simulink model "ROPOD_4Wheel_TdistZMPC_cntr"  (R2017b)
settings: Solver=FixedStepAuto  StartTime=0.0  StopTime=Inf  FixedStep=Ts  RelTol=1e-3
PreLoadFcn:
  | cd /home/robocup/RoPod/Force_dist_ZMPC_ROS
  | init_model
InitFcn:
  | cd /home/robocup/RoPod/Force_dist_ZMPC_ROS
  | init_model
values from neighbouring files (symbols this model uses):
  b_cx = 36.5    [RoPod_parameters.mat]
  b_cy = 36.5    [RoPod_parameters.mat]
  Fd_max = 70    [RoPod_parameters.mat]
  Fd_min = 20    [RoPod_parameters.mat]
  FFtheta_intia = 0    [init_model.m]
  FFxy_mass = 80    [init_model.m]
  Fr_max = 100    [RoPod_parameters.mat]
  Fr_min = -100    [RoPod_parameters.mat]
  k_cx = 1713    [RoPod_parameters.mat]
  k_cy = 4489    [RoPod_parameters.mat]
  max_hw_tau = 7.0    (= 7)    [init_model.m]
  Nwheels = 4    [init_model.m]
  pivot_offs_sws = [2.21 1.873 2.001 3.508]    [init_model.m]
  SW_COM1_ENABLE1 = hex2dec('0001')    [init_model.m]
  SW_COM1_ENABLE2 = hex2dec('0002')    [init_model.m]
  SW_COM1_MODE_TORQUE = bitshift(hex2dec('0000'),2)    [init_model.m]
  SW_COM1_MODE_VELOCITY = bitshift(hex2dec('0002'),2)    [init_model.m]
  SW_COM1_USE_TS = hex2dec('8000')    [init_model.m]
  sw_tau_2_curr = 1/motor_physical_parameters.torqueconstant.value    [init_model.m]
  Taucompfactor = 2.0    (= 2)    [init_model.m]
  Tinit = 1*Tslot    [init_model.m]
  Ts = 0.001    [init_model.m]
  Ts_MPC = 0.001    [init_model.m]
  Tsp = 1    [init_model.m]
  xA = [1 -1 0 0 0 0 0.0206696424966 -0.0206696424966 0 0 0.0298227588181 -0.0298227588181 ... (4080 elements, 102x40)]    [ZMPCx_parameters.mat]
  xBd_dis = [1.12932348493e-06 0.000225071897401 0 0]    [ZMPCx_parameters.mat]
  xF = [0 0 0 0 0 0 0 0 0 0 0 0 ... (80 elements, 20x4)]    [ZMPCx_parameters.mat]
  xH = [20 0 0 0 0 0 0 0 0 0 0 0 ... (1600 elements, 40x40)]    [ZMPCx_parameters.mat]
  xPhi = [0.995143909015 -0.967809158823 0 0 0.980727027327 -1.91066813489 0 0 0.957042868744 -2.81984596436 0 0 ... (320 elements, 80x4)]    [ZMPCx_parameters.mat]
  xrho = 144000    [ZMPCx_parameters.mat]
  xW = [0 0 -4300 4300 0 0 -4211.12053726 4211.12053726 0 0 -4082.88267435 4082.88267435 ... (328 elements, 82x4)]    [ZMPCx_parameters.mat]
  yA = [1 -1 0 0 0 0 0.0146537039222 -0.0146537039222 0 0 0.0255124036215 -0.0255124036215 ... (4080 elements, 102x40)]    [ZMPCy_parameters.mat]
  yBd_dis = [1.24492522358e-06 0.000248362591603 0 0]    [ZMPCy_parameters.mat]
  yF = [0.00191047141222 0.00156448969707 0.00119761396088 0.000813779538874 0.00041715000072 1.20724055612e-05 -0.00039696993291 -0.000805406662726 -0.00120863105559 -0.00160205155743 -0.00198114365531 -0.00234150147928 ... (80 elements, 20x4)]    [ZMPCy_parameters.mat]
  yH = [2.00000002801 0 2.31602594113e-08 0 1.80085634996e-08 0 1.26053094289e-08 0 7.00898668547e-09 0 1.2808124932e-09 0 ... (1600 elements, 40x40)]    [ZMPCy_parameters.mat]
  yPhi = [0.994411530671 -1.11489967371 0 0 0.977778317439 -2.20691845877 0 0 0.950389393786 -3.2640842851 0 0 ... (320 elements, 80x4)]    [ZMPCy_parameters.mat]
  yrho = 10000    [ZMPCy_parameters.mat]
  yW = [0 0 -4489 4489 0 0 -4423.21952309 4423.21952309 0 0 -4308.69434324 4308.69434324 ... (328 elements, 82x4)]    [ZMPCy_parameters.mat]
undefined symbols (not defined in the file or in its folder): DiscIntNeverNeededParam, Pose, ropod_kinmodel_param, Twist, Wrench
libraries: cstblocks x85, robotlib x60, simulink x41, SOEM_EtherCAT_Lib x5, robotcorelib x1
(part 1 of 6)
PreSaveFcn:
  | cd /home/robocup/RoPod/Force_dist_ZMPC_ROS
  | init_model
settings Model: Creator=cesar  LastModifiedBy=root
settings OptimizationCC: PassReuseOutputArgsAs=Individual arguments  MaxStackSize=64
settings DebuggingCC: ParameterTunabilityLossMsg=error
settings HardwareCC: ProdBitPerLong=64  ProdHWDeviceType=Intel->x86-64 (Linux 64)  TargetBitPerLong=64  TargetBitPerPointer=64  TargetBitPerSizeT=64  TargetBitPerPtrDiffT=64  TargetLargestAtomicFloat=Float  TargetIntDivRoundTo=Zero  TargetEndianess=LittleEndian  TargetWordSize=64  TargetHWDeviceType=Intel->x86-64 (Linux 64)
settings SFSimCC: MATLABDynamicMemAlloc=off
settings RTWCC: SystemTargetFile=ert.tlc  HardwareBoard=Robot Operating System (ROS)  TemplateMakefile=ert_default_tmf  GenerateReport=on  RTWVerbose=off  CustomInclude=/usr/local/include/soem  CustomLibrary=/usr/local/lib/libsoem.so  Toolchain=Catkin  BuildConfiguration=Faster Runs  IncludeHyperlinkInReport=on  LaunchReport=on  TargetLang=C++  GenerateTraceInfo=on  GenerateTraceReport=on  GenerateTraceReportSl=on  GenerateTraceReportSf=on  GenerateTraceReportEml=on
settings CodeAppCC: ForceParamTrailComments=on  IgnoreCustomStorageClasses=off  OperatorAnnotations=on  SimulinkDataObjDesc=on  SFDataObjDesc=on  InsertBlockDesc=on
settings ERTTargetCC: SupportNonInlinedSFcns=on  SupportVariableSizeSignals=on

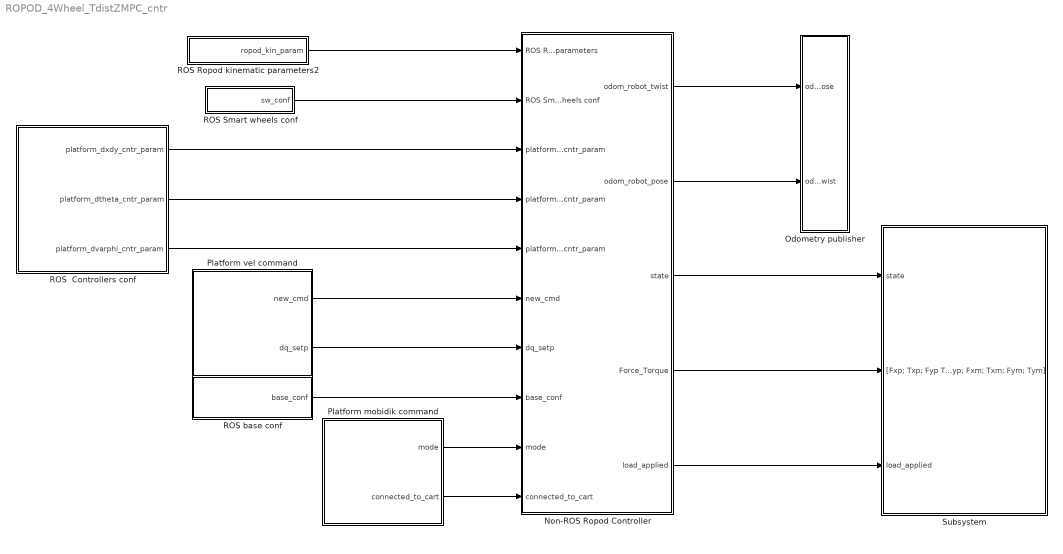
== system ROPOD_4Wheel_TdistZMPC_cntr ==
  Non-ROS Ropod Controller : Subsystem
  Odometry publisher : Subsystem
  Platform mobidik command : Subsystem
  Platform vel command : Subsystem
  ROS  Controllers conf : Subsystem
  ROS Ropod kinematic parameters2 : Subsystem
  ROS Smart wheels conf : Subsystem
  ROS base conf : Subsystem
  Subsystem : Subsystem
  wires:
  ROS Ropod kinematic parameters2/1(ropod_kin_param) -> Non-ROS Ropod Controller/1(ROS Ropod kinematic parameters)
  ROS Smart wheels conf/1(sw_conf) -> Non-ROS Ropod Controller/2(ROS Smart wheels conf)
  ROS  Controllers conf/1(platform_dxdy_cntr_param) -> Non-ROS Ropod Controller/3(platform_dxdy_cntr_param)
  ROS  Controllers conf/2(platform_dtheta_cntr_param) -> Non-ROS Ropod Controller/4(platform_dtheta_cntr_param)
  ROS  Controllers conf/3(platform_dvarphi_cntr_param) -> Non-ROS Ropod Controller/5(platform_dvarphi_cntr_param)
  Platform vel command/1(new_cmd) -> Non-ROS Ropod Controller/6(new_cmd)
  Platform vel command/2(dq_setp) -> Non-ROS Ropod Controller/7(dq_setp)
  ROS base conf/1(base_conf) -> Non-ROS Ropod Controller/8(base_conf)
  Non-ROS Ropod Controller/1(odom_robot_twist) -> Odometry publisher/1(odom_pose)
  Non-ROS Ropod Controller/2(odom_robot_pose) -> Odometry publisher/2(odom_twist)
  Non-ROS Ropod Controller/3(state) -> Subsystem/1(state)
  Non-ROS Ropod Controller/4(Force_Torque) -> Subsystem/2("[Fxp; Txp; Fyp Typ; Fxm; Txm; Fym; Tym] ")
  Platform mobidik command/1(mode) -> Non-ROS Ropod Controller/9(mode)
  Platform mobidik command/2(connected_to_cart) -> Non-ROS Ropod Controller/10(connected_to_cart)
  Non-ROS Ropod Controller/5(load_applied) -> Subsystem/3(load_applied)

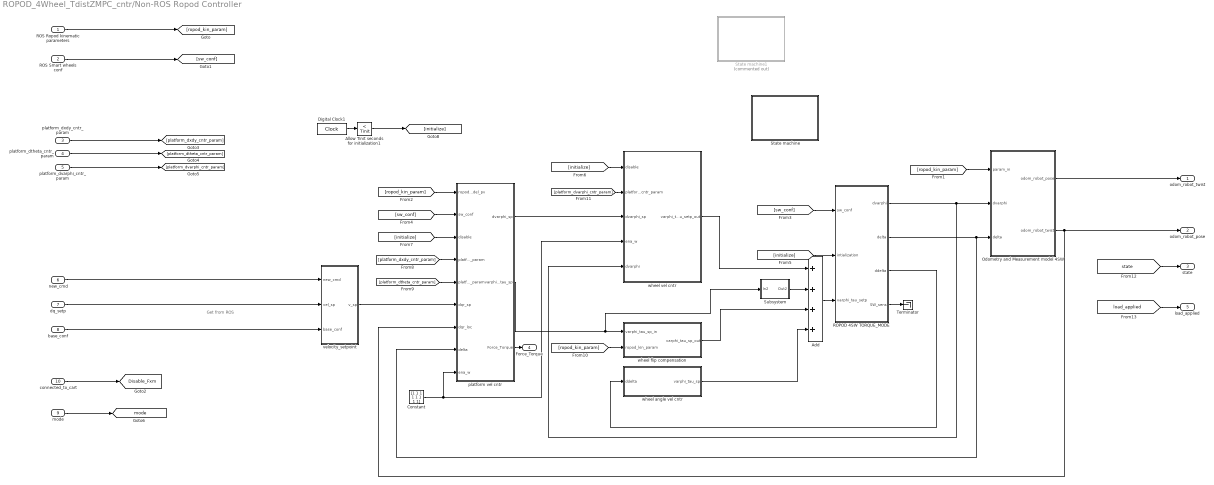
== system ROPOD_4Wheel_TdistZMPC_cntr/Non-ROS Ropod Controller ==
  note: Get from ROS
  ROS Ropod kinematic parameters : Inport
  ROS Smart wheels conf : Inport  Port=2
  platform_dxdy_cntr_param : Inport  Port=3
  platform_dtheta_cntr_param : Inport  Port=4
  platform_dvarphi_cntr_param : Inport  Port=5
  new_cmd : Inport  Port=6
  dq_setp : Inport  Port=7
  base_conf : Inport  Port=8
  mode : Inport  Port=9
  connected_to_cart : Inport  Port=10
  Add : Sum  Inputs=++++
  Allow Tinit seconds for initialization1 : simulink/Logic and Bit Operations/Compare To Constant  relop=<  const=Tinit  OutDataTypeStr=boolean
  Constant : Constant  Value=[1 1 1 1 1 1 1 1]
  Digital Clock1 : DigitalClock  SampleTime=Ts
  Odometry and Measurement model 4SW : Subsystem
  ROPOD 4SW TORQUE_MODE : Subsystem
  State machine : Subsystem
  State machine1 : Subsystem  Commented=on
  Subsystem : Subsystem
  Terminator : Terminator
  platform vel cntr : Subsystem
  velocity_setpoint : Subsystem
  wheel angle vel cntr : Subsystem
  wheel flip compensation : Subsystem
  wheel vel cntr : Subsystem
  odom_robot_twist : Outport
  odom_robot_pose : Outport  Port=2
  state : Outport  Port=3
  Force_Torque : Outport  Port=4
  load_applied : Outport  Port=5
  tag scope: Disable_Fxm=global, mode=global
  wires:
  [sw_conf] -> ROPOD 4SW TORQUE_MODE/1(sw_conf)
  ROPOD 4SW TORQUE_MODE/3(ddelta) -> wheel angle vel cntr/1(ddelta)
  [initialize] -> wheel vel cntr/1(disable)
  base_conf/1 -> velocity_setpoint/3(base_conf)
  Digital Clock1/1 -> Allow Tinit seconds for initialization1/1
  [sw_conf] -> platform vel cntr/2(sw_conf)
  [platform_dvarphi_cntr_param] -> wheel vel cntr/2(platform_dxdy_cntr_param)
  wheel angle vel cntr/1(varphi_tau_sp) -> Add/4
  ROPOD 4SW TORQUE_MODE/2(delta) -> Odometry and Measurement model 4SW/3(delta), platform vel cntr/8(delta)
  [platform_dtheta_cntr_param] -> platform vel cntr/5(platform_dtheta_cntr_param)
  platform vel cntr/2(varphi_tau_sp) -> Subsystem/1(In2), wheel flip compensation/1(varphi_tau_sp_in)
  Add/1 -> ROPOD 4SW TORQUE_MODE/3(varphi_tau_setp)
  [platform_dxdy_cntr_param] -> platform vel cntr/4(platform_dxdy_cntr_param)
  [ropod_kin_param] -> platform vel cntr/1(ropod_kinmodel_pv)
  velocity_setpoint/1(v_sp) -> platform vel cntr/6(dqr_sp)
  wheel flip compensation/1(varphi_tau_sp_out) -> Add/3
  ROS Smart wheels conf/1 -> [sw_conf]
  platform_dvarphi_cntr_param/1 -> [platform_dvarphi_cntr_param]
  Odometry and Measurement model 4SW/1(odom_robot_pose) -> odom_robot_twist/1
  [ropod_kin_param] -> Odometry and Measurement model 4SW/1(param_in)
  [initialize] -> platform vel cntr/3(disable)
  ROPOD 4SW TORQUE_MODE/4(SW_sens) -> Terminator/1
  platform_dxdy_cntr_param/1 -> [platform_dxdy_cntr_param]
  ROS Ropod kinematic parameters/1 -> [ropod_kin_param]
  [initialize] -> ROPOD 4SW TORQUE_MODE/2(intialization)
  [ropod_kin_param] -> wheel flip compensation/2(ropod_kin_param)
  platform vel cntr/1(dvarphi_sp) -> wheel vel cntr/3(dvarphi_sp)
  Odometry and Measurement model 4SW/2(odom_robot_twist) -> odom_robot_pose/1, platform vel cntr/7(dqr_loc)
  ROPOD 4SW TORQUE_MODE/1(dvarphi) -> Odometry and Measurement model 4SW/2(dvarphi), wheel vel cntr/5(dvarphi)
  platform_dtheta_cntr_param/1 -> [platform_dtheta_cntr_param]
  new_cmd/1 -> velocity_setpoint/1(new_cmd)
  dq_setp/1 -> velocity_setpoint/2(vel_sp)
  Constant/1 -> wheel vel cntr/4(ena_w), platform vel cntr/9(ena_w)
  Allow Tinit seconds for initialization1/1 -> [initialize]
  wheel vel cntr/1(varphi_tau_setp_out) -> Add/1
  Subsystem/1(Out2) -> Add/2
  connected_to_cart/1 -> [Disable_Fxm]
  mode/1 -> [mode]
  [state] -> state/1
  platform vel cntr/3(Force_Torque) -> Force_Torque/1
  [load_applied] -> load_applied/1

== system ROPOD_4Wheel_TdistZMPC_cntr/Odometry publisher ==
  odom_pose : Inport
  odom_twist : Inport  Port=2
  Blank Message : robotlib/Blank Message  SourceLibraryInfo=This block requires Robotics System Toolbox  messageType=nav_msgs/Odometry  SampleTime=-1
      settings: SourceProductBaseCode=RO
  Bus Assignment : BusAssignment  AssignedSignals=Pose.Pose.Position.X,Pose.Pose.Position.Y,Pose.Pose.Position.Z,Pose.Pose.Orientation.W,Pose.Pose.Orientation.X,Pose.Pose.Orientation.Y,Pose.Pose.Orientation.Z,Twist.Twist.Linear.X,Twist.Twist.Linear.Y,Twist.Twist.Linear.Z,Twist.Twist.Angular.X,Twist.Twist.Angular.Y,Twist.Twist.Angular.Z
  Constant{,1..5} (6 alike) : Constant  Value=0
  Coordinate Transformation Conversion : robotcorelib/Coordinate Transformation Conversion  InputRepresentation=Euler Angles  InputEulerSequence=XYZ  ShowTrVecInputPort=on  OutputRepresentation=Quaternion  OutputEulerSequence=ZYX  ShowTrVecOutputPort=on  SimulateUsing=Code generation
      settings: SourceProductBaseCode=RO
  Demux : Demux  Outputs=3
  Demux1 : Demux
  Demux2 : Demux  Outputs=3
  Mux : Mux  Inputs=3
  Publish : robotlib/Publish  SourceLibraryInfo=This block requires Robotics System Toolbox  topicSource=Specify your own  topic=/odom_incomplete  messageType=nav_msgs/Odometry  messageQueueLength=1
      settings: SourceProductBaseCode=RO
  Rate Transition : RateTransition  OutPortSampleTime=Ts_rost
  wires:
  Demux2/2 -> Bus Assignment/10
  Bus Assignment/1 -> Rate Transition/1
  Constant2/1 -> Mux/2
  Constant3/1 -> Bus Assignment/11
  Constant/1 -> Bus Assignment/4
  Constant4/1 -> Bus Assignment/12
  Demux2/1 -> Bus Assignment/9
  Coordinate Transformation Conversion/1 -> Demux1/1
  Constant5/1 -> Bus Assignment/13
  Demux/3 -> Mux/3
  Mux/1 -> Coordinate Transformation Conversion/1
  odom_pose/1 -> Demux/1
  Demux/1 -> Bus Assignment/2
  Constant1/1 -> Mux/1
  odom_twist/1 -> Demux2/1
  Demux/2 -> Bus Assignment/3
  Blank Message/1 -> Bus Assignment/1
  Demux2/3 -> Bus Assignment/14
  Rate Transition/1 -> Publish/1
  Demux1/1 -> Bus Assignment/5
  Demux1/2 -> Bus Assignment/6
  Demux1/3 -> Bus Assignment/7
  Demux1/4 -> Bus Assignment/8

== system ROPOD_4Wheel_TdistZMPC_cntr/Platform mobidik command ==
  Bus Selector : BusSelector  OutputSignals=Data
  Bus Selector1 : BusSelector  OutputSignals=Data
  Subscribe1 : robotlib/Subscribe  SourceLibraryInfo=This block requires Robotics System Toolbox  topicSource=Specify your own  topic=/ropod/Set_LLCmode  messageType=std_msgs/UInt16  sampleTime=Ts_rost  messageQueueLength=5
      settings: SourceProductBaseCode=RO
  Subscribe2 : robotlib/Subscribe  SourceLibraryInfo=This block requires Robotics System Toolbox  topicSource=Specify your own  topic=/route_navigation/set_load_attached  messageType=std_msgs/Bool  sampleTime=Ts_rost  messageQueueLength=5
      settings: SourceProductBaseCode=RO
  Terminator : Terminator
  Terminator1 : Terminator
  mode : Outport
  connected_to_cart : Outport  Port=2
  wires:
  Subscribe2/2 -> Bus Selector/1
  Subscribe1/1 -> Terminator/1
  Subscribe2/1 -> Terminator1/1
  Bus Selector/1 -> connected_to_cart/1  "<Data>"
  Subscribe1/2 -> Bus Selector1/1
  Bus Selector1/1 -> mode/1  "<Data>"

== system ROPOD_4Wheel_TdistZMPC_cntr/Platform vel command ==
  Bus Selector : BusSelector  OutputSignals=Linear.X,Linear.Y,Angular.Z
  Mux : Mux  Inputs=3.
  Subscribe1 : robotlib/Subscribe  SourceLibraryInfo=This block requires Robotics System Toolbox  topicSource=Specify your own  topic=/cmd_vel  messageType=geometry_msgs/Twist  sampleTime=Ts_rost  messageQueueLength=5
      settings: SourceProductBaseCode=RO
  new_cmd : Outport
  dq_setp : Outport  Port=2
  wires:
  Subscribe1/1 -> new_cmd/1
  Subscribe1/2 -> Bus Selector/1
  Bus Selector/1 -> Mux/1  "<X>"
  Bus Selector/2 -> Mux/2  "<Y>"
  Bus Selector/3 -> Mux/3  "<Z>"
  Mux/1 -> dq_setp/1

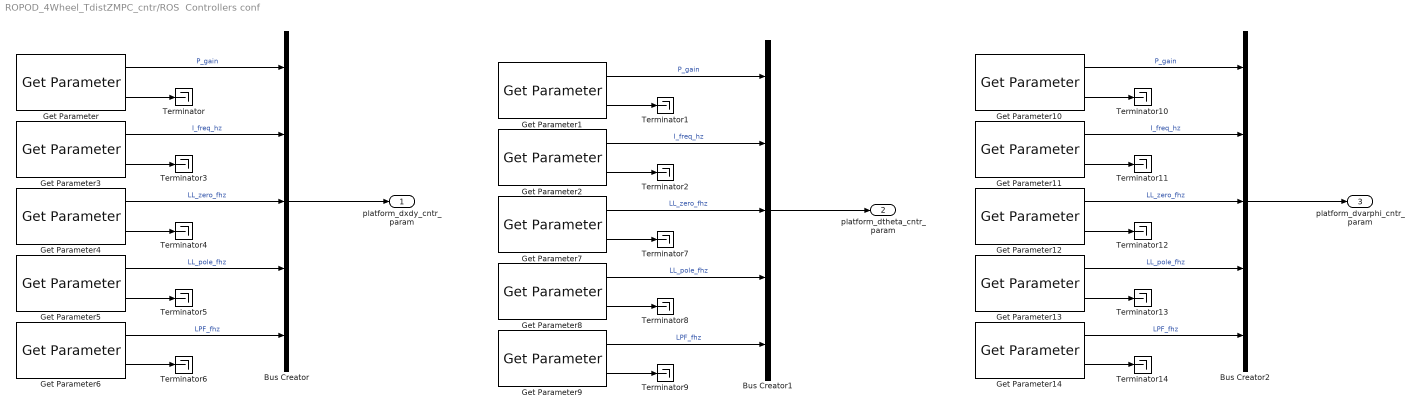
== system ROPOD_4Wheel_TdistZMPC_cntr/ROS  Controllers conf ==
  Bus Creator : BusCreator  Inputs=5
  Bus Creator1 : BusCreator  Inputs=5
  Bus Creator2 : BusCreator  Inputs=5
  Get Parameter : robotlib/Get Parameter  SourceLibraryInfo=This block requires Robotics System Toolbox  ParameterSource=Specify your own  ParameterName=/platform_dxdy_cntr/Kgain  ParameterType=double  ParameterMaxArrayLength=16  ParameterInitialValue=K_gain_dxdy_cntr  SampleTime=Tsp  ShowErrorCodeOutput=on  ModelName=ROPOD_4Wheel_TdistZMPC_cntr  BlockId=ParamGet_ROPOD_4Wheel_TdistZMPC_cntr_2716
      settings: SourceProductName=Robotics System Toolbox  SourceProductBaseCode=RO
  Get Parameter1 : robotlib/Get Parameter  SourceLibraryInfo=This block requires Robotics System Toolbox  ParameterSource=Specify your own  ParameterName=/platform_dtheta_cntr/Kgain  ParameterType=double  ParameterMaxArrayLength=16  ParameterInitialValue=K_gain_dtheta_cntr  SampleTime=Tsp  ShowErrorCodeOutput=on  ModelName=ROPOD_4Wheel_TdistZMPC_cntr  BlockId=ParamGet_ROPOD_4Wheel_TdistZMPC_cntr_2919
      settings: SourceProductName=Robotics System Toolbox  SourceProductBaseCode=RO
  Get Parameter10 : robotlib/Get Parameter  SourceLibraryInfo=This block requires Robotics System Toolbox  ParameterSource=Specify your own  ParameterName=/platform_dvarphi_cntr/Kgain  ParameterType=double  ParameterMaxArrayLength=16  ParameterInitialValue=K_gain_dvarphi_cntr  SampleTime=Tsp  ShowErrorCodeOutput=on  ModelName=ROPOD_4Wheel_TdistZMPC_cntr  BlockId=ParamGet_ROPOD_4Wheel_TdistZMPC_cntr_2931
      settings: SourceProductName=Robotics System Toolbox  SourceProductBaseCode=RO
  Get Parameter11 : robotlib/Get Parameter  SourceLibraryInfo=This block requires Robotics System Toolbox  ParameterSource=Specify your own  ParameterName=/platform_dvarphi_cntr/I_fhz  ParameterType=double  ParameterMaxArrayLength=16  ParameterInitialValue=I_fhz_dvarphi_cntr  SampleTime=Tsp  ShowErrorCodeOutput=on  ModelName=ROPOD_4Wheel_TdistZMPC_cntr  BlockId=ParamGet_ROPOD_4Wheel_TdistZMPC_cntr_2932
      settings: SourceProductName=Robotics System Toolbox  SourceProductBaseCode=RO
  Get Parameter12 : robotlib/Get Parameter  SourceLibraryInfo=This block requires Robotics System Toolbox  ParameterSource=Specify your own  ParameterName=/platform_dvarphi_cntr/LL_wz_fhz  ParameterType=double  ParameterMaxArrayLength=16  ParameterInitialValue=LL_wz_fhz_dvarphi_cntr  SampleTime=Tsp  ShowErrorCodeOutput=on  ModelName=ROPOD_4Wheel_TdistZMPC_cntr  BlockId=ParamGet_ROPOD_4Wheel_TdistZMPC_cntr_2933
      settings: SourceProductName=Robotics System Toolbox  SourceProductBaseCode=RO
  Get Parameter13 : robotlib/Get Parameter  SourceLibraryInfo=This block requires Robotics System Toolbox  ParameterSource=Specify your own  ParameterName=/platform_dvarphi_cntr/LL_wp_fhz  ParameterType=double  ParameterMaxArrayLength=16  ParameterInitialValue=LL_wp_fhz_dvarphi_cntr  SampleTime=Tsp  ShowErrorCodeOutput=on  ModelName=ROPOD_4Wheel_TdistZMPC_cntr  BlockId=ParamGet_ROPOD_4Wheel_TdistZMPC_cntr_2934
      settings: SourceProductName=Robotics System Toolbox  SourceProductBaseCode=RO
  Get Parameter14 : robotlib/Get Parameter  SourceLibraryInfo=This block requires Robotics System Toolbox  ParameterSource=Specify your own  ParameterName=/platform_dvarphi_cntr/LPF_fhz  ParameterType=double  ParameterMaxArrayLength=16  ParameterInitialValue=LPF_fhz_dvarphi_cntr  SampleTime=Tsp  ShowErrorCodeOutput=on  ModelName=ROPOD_4Wheel_TdistZMPC_cntr  BlockId=ParamGet_ROPOD_4Wheel_TdistZMPC_cntr_2935
      settings: SourceProductName=Robotics System Toolbox  SourceProductBaseCode=RO
  Get Parameter2 : robotlib/Get Parameter  SourceLibraryInfo=This block requires Robotics System Toolbox  ParameterSource=Specify your own  ParameterName=/platform_dtheta_cntr/I_fhz  ParameterType=double  ParameterMaxArrayLength=16  ParameterInitialValue=I_fhz_dtheta_cntr  SampleTime=Tsp  ShowErrorCodeOutput=on  ModelName=ROPOD_4Wheel_TdistZMPC_cntr  BlockId=ParamGet_ROPOD_4Wheel_TdistZMPC_cntr_2920
      settings: SourceProductName=Robotics System Toolbox  SourceProductBaseCode=RO
  Get Parameter3 : robotlib/Get Parameter  SourceLibraryInfo=This block requires Robotics System Toolbox  ParameterSource=Specify your own  ParameterName=/platform_dxdy_cntr/I_fhz  ParameterType=double  ParameterMaxArrayLength=16  ParameterInitialValue=I_fhz_dxdy_cntr  SampleTime=Tsp  ShowErrorCodeOutput=on  ModelName=ROPOD_4Wheel_TdistZMPC_cntr  BlockId=ParamGet_ROPOD_4Wheel_TdistZMPC_cntr_2898
      settings: SourceProductName=Robotics System Toolbox  SourceProductBaseCode=RO
  Get Parameter4 : robotlib/Get Parameter  SourceLibraryInfo=This block requires Robotics System Toolbox  ParameterSource=Specify your own  ParameterName=/platform_dxdy_cntr/LL_wz_fhz  ParameterType=double  ParameterMaxArrayLength=16  ParameterInitialValue=LL_wz_fhz_dxdy_cntr  SampleTime=Tsp  ShowErrorCodeOutput=on  ModelName=ROPOD_4Wheel_TdistZMPC_cntr  BlockId=ParamGet_ROPOD_4Wheel_TdistZMPC_cntr_2900
      settings: SourceProductName=Robotics System Toolbox  SourceProductBaseCode=RO
  Get Parameter5 : robotlib/Get Parameter  SourceLibraryInfo=This block requires Robotics System Toolbox  ParameterSource=Specify your own  ParameterName=/platform_dxdy_cntr/LL_wp_fhz  ParameterType=double  ParameterMaxArrayLength=16  ParameterInitialValue=LL_wp_fhz_dxdy_cntr  SampleTime=Tsp  ShowErrorCodeOutput=on  ModelName=ROPOD_4Wheel_TdistZMPC_cntr  BlockId=ParamGet_ROPOD_4Wheel_TdistZMPC_cntr_2902
      settings: SourceProductName=Robotics System Toolbox  SourceProductBaseCode=RO
  Get Parameter6 : robotlib/Get Parameter  SourceLibraryInfo=This block requires Robotics System Toolbox  ParameterSource=Specify your own  ParameterName=/platform_dxdy_cntr/LPF_fhz  ParameterType=double  ParameterMaxArrayLength=16  ParameterInitialValue=LPF_fhz_dxdy_cntr  SampleTime=Tsp  ShowErrorCodeOutput=on  ModelName=ROPOD_4Wheel_TdistZMPC_cntr  BlockId=ParamGet_ROPOD_4Wheel_TdistZMPC_cntr_2903
      settings: SourceProductName=Robotics System Toolbox  SourceProductBaseCode=RO
  Get Parameter7 : robotlib/Get Parameter  SourceLibraryInfo=This block requires Robotics System Toolbox  ParameterSource=Specify your own  ParameterName=/platform_dtheta_cntr/LL_wz_fhz  ParameterType=double  ParameterMaxArrayLength=16  ParameterInitialValue=LL_wz_fhz_dtheta_cntr  SampleTime=Tsp  ShowErrorCodeOutput=on  ModelName=ROPOD_4Wheel_TdistZMPC_cntr  BlockId=ParamGet_ROPOD_4Wheel_TdistZMPC_cntr_2921
      settings: SourceProductName=Robotics System Toolbox  SourceProductBaseCode=RO
  Get Parameter8 : robotlib/Get Parameter  SourceLibraryInfo=This block requires Robotics System Toolbox  ParameterSource=Specify your own  ParameterName=/platform_dtheta_cntr/LL_wp_fhz  ParameterType=double  ParameterMaxArrayLength=16  ParameterInitialValue=LL_wp_fhz_dtheta_cntr  SampleTime=Tsp  ShowErrorCodeOutput=on  ModelName=ROPOD_4Wheel_TdistZMPC_cntr  BlockId=ParamGet_ROPOD_4Wheel_TdistZMPC_cntr_2922
      settings: SourceProductName=Robotics System Toolbox  SourceProductBaseCode=RO
  Get Parameter9 : robotlib/Get Parameter  SourceLibraryInfo=This block requires Robotics System Toolbox  ParameterSource=Specify your own  ParameterName=/platform_dtheta_cntr/LPF_fhz  ParameterType=double  ParameterMaxArrayLength=16  ParameterInitialValue=LPF_fhz_dtheta_cntr  SampleTime=Tsp  ShowErrorCodeOutput=on  ModelName=ROPOD_4Wheel_TdistZMPC_cntr  BlockId=ParamGet_ROPOD_4Wheel_TdistZMPC_cntr_2923
      settings: SourceProductName=Robotics System Toolbox  SourceProductBaseCode=RO
  Terminator{,1..14} (15 alike) : Terminator
  platform_dxdy_cntr_param : Outport
  platform_dtheta_cntr_param : Outport  Port=2
  platform_dvarphi_cntr_param : Outport  Port=3
  wires:
  Get Parameter/2 -> Terminator/1
  Get Parameter5/1 -> Bus Creator/4  "LL_pole_fhz"
  Get Parameter6/1 -> Bus Creator/5  "LPF_fhz"
  Bus Creator/1 -> platform_dxdy_cntr_param/1
  Get Parameter3/1 -> Bus Creator/2  "I_freq_hz"
  Get Parameter4/1 -> Bus Creator/3  "LL_zero_fhz"
  Get Parameter/1 -> Bus Creator/1  "P_gain"
  Get Parameter3/2 -> Terminator3/1
  Get Parameter4/2 -> Terminator4/1
  Get Parameter5/2 -> Terminator5/1
  Get Parameter6/2 -> Terminator6/1
  Get Parameter8/1 -> Bus Creator1/4  "LL_pole_fhz"
  Get Parameter9/2 -> Terminator9/1
  Get Parameter2/1 -> Bus Creator1/2  "I_freq_hz"
  Get Parameter8/2 -> Terminator8/1
  Bus Creator1/1 -> platform_dtheta_cntr_param/1
  Get Parameter2/2 -> Terminator2/1
  Get Parameter7/1 -> Bus Creator1/3  "LL_zero_fhz"
  Get Parameter7/2 -> Terminator7/1
  Get Parameter1/1 -> Bus Creator1/1  "P_gain"
  Get Parameter1/2 -> Terminator1/1
  Get Parameter9/1 -> Bus Creator1/5  "LPF_fhz"
  Get Parameter10/2 -> Terminator10/1
  Get Parameter13/2 -> Terminator13/1
  Get Parameter14/2 -> Terminator14/1
  Get Parameter11/1 -> Bus Creator2/2  "I_freq_hz"
  Get Parameter10/1 -> Bus Creator2/1  "P_gain"
  Get Parameter11/2 -> Terminator11/1
  Get Parameter13/1 -> Bus Creator2/4  "LL_pole_fhz"
  Bus Creator2/1 -> platform_dvarphi_cntr_param/1
  Get Parameter12/2 -> Terminator12/1
  Get Parameter12/1 -> Bus Creator2/3  "LL_zero_fhz"
  Get Parameter14/1 -> Bus Creator2/5  "LPF_fhz"

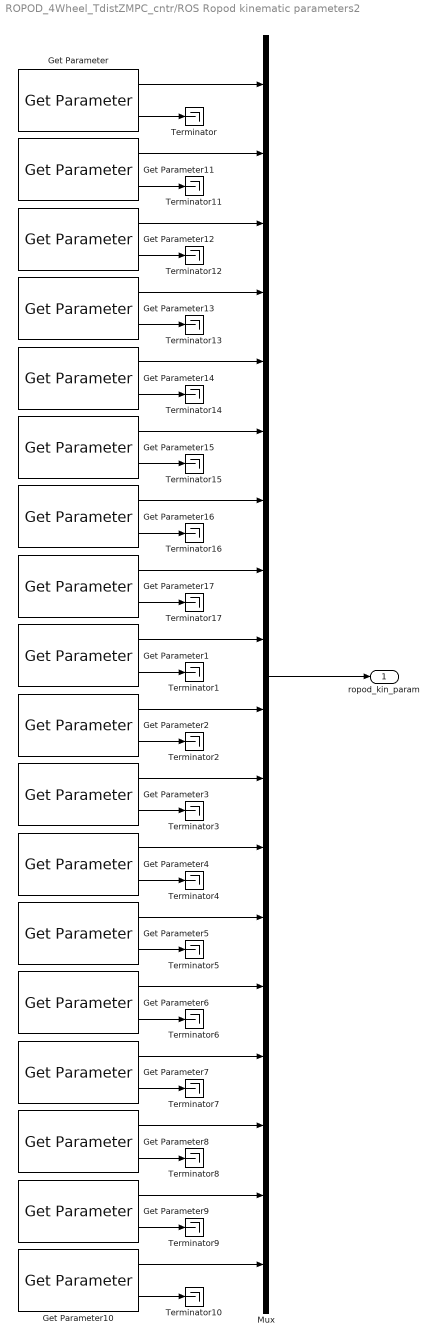
== system ROPOD_4Wheel_TdistZMPC_cntr/ROS Ropod kinematic parameters2 ==
  Get Parameter : robotlib/Get Parameter  SourceLibraryInfo=This block requires Robotics System Toolbox  ParameterSource=Specify your own  ParameterName=/base_kin_model/r_wL_SW1  ParameterType=double  ParameterMaxArrayLength=16  ParameterInitialValue=ropod_kinmodel_param.r_w(1)  SampleTime=Tsp  ShowErrorCodeOutput=on  ModelName=ROPOD_4Wheel_TdistZMPC_cntr  BlockId=ParamGet_ROPOD_4Wheel_TdistZMPC_cntr_2173
      settings: SourceProductName=Robotics System Toolbox  SourceProductBaseCode=RO
  Get Parameter1 : robotlib/Get Parameter  SourceLibraryInfo=This block requires Robotics System Toolbox  ParameterSource=Specify your own  ParameterName=/base_kin_model/s_w  ParameterType=double  ParameterMaxArrayLength=16  ParameterInitialValue=ropod_kinmodel_param.s_w  SampleTime=Tsp  ShowErrorCodeOutput=on  ModelName=ROPOD_4Wheel_TdistZMPC_cntr  BlockId=ParamGet_ROPOD_4Wheel_TdistZMPC_cntr_2174
      settings: SourceProductName=Robotics System Toolbox  SourceProductBaseCode=RO
  Get Parameter10 : robotlib/Get Parameter  SourceLibraryInfo=This block requires Robotics System Toolbox  ParameterSource=Specify your own  ParameterName=/base_kin_model/ypos_SW4  ParameterType=double  ParameterMaxArrayLength=16  ParameterInitialValue=ropod_kinmodel_param.C_SW(8)  SampleTime=Tsp  ShowErrorCodeOutput=on  ModelName=ROPOD_4Wheel_TdistZMPC_cntr  BlockId=ParamGet_ROPOD_4Wheel_TdistZMPC_cntr_2175
      settings: SourceProductName=Robotics System Toolbox  SourceProductBaseCode=RO
  Get Parameter11 : robotlib/Get Parameter  SourceLibraryInfo=This block requires Robotics System Toolbox  ParameterSource=Specify your own  ParameterName=/base_kin_model/r_wR_SW1  ParameterType=double  ParameterMaxArrayLength=16  ParameterInitialValue=ropod_kinmodel_param.r_w(2)  SampleTime=Tsp  ShowErrorCodeOutput=on  ModelName=ROPOD_4Wheel_TdistZMPC_cntr  BlockId=ParamGet_ROPOD_4Wheel_TdistZMPC_cntr_2176
      settings: SourceProductName=Robotics System Toolbox  SourceProductBaseCode=RO
  Get Parameter12 : robotlib/Get Parameter  SourceLibraryInfo=This block requires Robotics System Toolbox  ParameterSource=Specify your own  ParameterName=/base_kin_model/r_wL_SW2  ParameterType=double  ParameterMaxArrayLength=16  ParameterInitialValue=ropod_kinmodel_param.r_w(3)  SampleTime=Tsp  ShowErrorCodeOutput=on  ModelName=ROPOD_4Wheel_TdistZMPC_cntr  BlockId=ParamGet_ROPOD_4Wheel_TdistZMPC_cntr_2177
      settings: SourceProductName=Robotics System Toolbox  SourceProductBaseCode=RO
  Get Parameter13 : robotlib/Get Parameter  SourceLibraryInfo=This block requires Robotics System Toolbox  ParameterSource=Specify your own  ParameterName=/base_kin_model/r_wR_SW2  ParameterType=double  ParameterMaxArrayLength=16  ParameterInitialValue=ropod_kinmodel_param.r_w(4)  SampleTime=Tsp  ShowErrorCodeOutput=on  ModelName=ROPOD_4Wheel_TdistZMPC_cntr  BlockId=ParamGet_ROPOD_4Wheel_TdistZMPC_cntr_2178
      settings: SourceProductName=Robotics System Toolbox  SourceProductBaseCode=RO
  Get Parameter14 : robotlib/Get Parameter  SourceLibraryInfo=This block requires Robotics System Toolbox  ParameterSource=Specify your own  ParameterName=/base_kin_model/r_wL_SW3  ParameterType=double  ParameterMaxArrayLength=16  ParameterInitialValue=ropod_kinmodel_param.r_w(5)  SampleTime=Tsp  ShowErrorCodeOutput=on  ModelName=ROPOD_4Wheel_TdistZMPC_cntr  BlockId=ParamGet_ROPOD_4Wheel_TdistZMPC_cntr_2179
      settings: SourceProductName=Robotics System Toolbox  SourceProductBaseCode=RO
  Get Parameter15 : robotlib/Get Parameter  SourceLibraryInfo=This block requires Robotics System Toolbox  ParameterSource=Specify your own  ParameterName=/base_kin_model/r_wR_SW3  ParameterType=double  ParameterMaxArrayLength=16  ParameterInitialValue=ropod_kinmodel_param.r_w(6)  SampleTime=Tsp  ShowErrorCodeOutput=on  ModelName=ROPOD_4Wheel_TdistZMPC_cntr  BlockId=ParamGet_ROPOD_4Wheel_TdistZMPC_cntr_2180
      settings: SourceProductName=Robotics System Toolbox  SourceProductBaseCode=RO
  Get Parameter16 : robotlib/Get Parameter  SourceLibraryInfo=This block requires Robotics System Toolbox  ParameterSource=Specify your own  ParameterName=/base_kin_model/r_wL_SW4  ParameterType=double  ParameterMaxArrayLength=16  ParameterInitialValue=ropod_kinmodel_param.r_w(7)  SampleTime=Tsp  ShowErrorCodeOutput=on  ModelName=ROPOD_4Wheel_TdistZMPC_cntr  BlockId=ParamGet_ROPOD_4Wheel_TdistZMPC_cntr_2181
      settings: SourceProductName=Robotics System Toolbox  SourceProductBaseCode=RO
  Get Parameter17 : robotlib/Get Parameter  SourceLibraryInfo=This block requires Robotics System Toolbox  ParameterSource=Specify your own  ParameterName=/base_kin_model/r_wR_SW4  ParameterType=double  ParameterMaxArrayLength=16  ParameterInitialValue=ropod_kinmodel_param.r_w(8)  SampleTime=Tsp  ShowErrorCodeOutput=on  ModelName=ROPOD_4Wheel_TdistZMPC_cntr  BlockId=ParamGet_ROPOD_4Wheel_TdistZMPC_cntr_2182
      settings: SourceProductName=Robotics System Toolbox  SourceProductBaseCode=RO
  Get Parameter2 : robotlib/Get Parameter  SourceLibraryInfo=This block requires Robotics System Toolbox  ParameterSource=Specify your own  ParameterName=/base_kin_model/d_w  ParameterType=double  ParameterMaxArrayLength=16  ParameterInitialValue=ropod_kinmodel_param.d_w  SampleTime=Tsp  ShowErrorCodeOutput=on  ModelName=ROPOD_4Wheel_TdistZMPC_cntr  BlockId=ParamGet_ROPOD_4Wheel_TdistZMPC_cntr_2183
      settings: SourceProductName=Robotics System Toolbox  SourceProductBaseCode=RO
  Get Parameter3 : robotlib/Get Parameter  SourceLibraryInfo=This block requires Robotics System Toolbox  ParameterSource=Specify your own  ParameterName=/base_kin_model/xpos_SW1  ParameterType=double  ParameterMaxArrayLength=16  ParameterInitialValue=ropod_kinmodel_param.C_SW(1)  SampleTime=Tsp  ShowErrorCodeOutput=on  ModelName=ROPOD_4Wheel_TdistZMPC_cntr  BlockId=ParamGet_ROPOD_4Wheel_TdistZMPC_cntr_2184
      settings: SourceProductName=Robotics System Toolbox  SourceProductBaseCode=RO
  Get Parameter4 : robotlib/Get Parameter  SourceLibraryInfo=This block requires Robotics System Toolbox  ParameterSource=Specify your own  ParameterName=/base_kin_model/ypos_SW1  ParameterType=double  ParameterMaxArrayLength=16  ParameterInitialValue=ropod_kinmodel_param.C_SW(2)  SampleTime=Tsp  ShowErrorCodeOutput=on  ModelName=ROPOD_4Wheel_TdistZMPC_cntr  BlockId=ParamGet_ROPOD_4Wheel_TdistZMPC_cntr_2185
      settings: SourceProductName=Robotics System Toolbox  SourceProductBaseCode=RO
  Get Parameter5 : robotlib/Get Parameter  SourceLibraryInfo=This block requires Robotics System Toolbox  ParameterSource=Specify your own  ParameterName=/base_kin_model/xpos_SW2  ParameterType=double  ParameterMaxArrayLength=16  ParameterInitialValue=ropod_kinmodel_param.C_SW(3)  SampleTime=Tsp  ShowErrorCodeOutput=on  ModelName=ROPOD_4Wheel_TdistZMPC_cntr  BlockId=ParamGet_ROPOD_4Wheel_TdistZMPC_cntr_2186
      settings: SourceProductName=Robotics System Toolbox  SourceProductBaseCode=RO
  Get Parameter6 : robotlib/Get Parameter  SourceLibraryInfo=This block requires Robotics System Toolbox  ParameterSource=Specify your own  ParameterName=/base_kin_model/ypos_SW2  ParameterType=double  ParameterMaxArrayLength=16  ParameterInitialValue=ropod_kinmodel_param.C_SW(4)  SampleTime=Tsp  ShowErrorCodeOutput=on  ModelName=ROPOD_4Wheel_TdistZMPC_cntr  BlockId=ParamGet_ROPOD_4Wheel_TdistZMPC_cntr_2187
      settings: SourceProductName=Robotics System Toolbox  SourceProductBaseCode=RO
  Get Parameter7 : robotlib/Get Parameter  SourceLibraryInfo=This block requires Robotics System Toolbox  ParameterSource=Specify your own  ParameterName=/base_kin_model/xpos_SW3  ParameterType=double  ParameterMaxArrayLength=16  ParameterInitialValue=ropod_kinmodel_param.C_SW(5)  SampleTime=Tsp  ShowErrorCodeOutput=on  ModelName=ROPOD_4Wheel_TdistZMPC_cntr  BlockId=ParamGet_ROPOD_4Wheel_TdistZMPC_cntr_2188
      settings: SourceProductName=Robotics System Toolbox  SourceProductBaseCode=RO
  Get Parameter8 : robotlib/Get Parameter  SourceLibraryInfo=This block requires Robotics System Toolbox  ParameterSource=Specify your own  ParameterName=/base_kin_model/ypos_SW3  ParameterType=double  ParameterMaxArrayLength=16  ParameterInitialValue=ropod_kinmodel_param.C_SW(6)  SampleTime=Tsp  ShowErrorCodeOutput=on  ModelName=ROPOD_4Wheel_TdistZMPC_cntr  BlockId=ParamGet_ROPOD_4Wheel_TdistZMPC_cntr_2189
      settings: SourceProductName=Robotics System Toolbox  SourceProductBaseCode=RO
  Get Parameter9 : robotlib/Get Parameter  SourceLibraryInfo=This block requires Robotics System Toolbox  ParameterSource=Specify your own  ParameterName=/base_kin_model/xpos_SW4  ParameterType=double  ParameterMaxArrayLength=16  ParameterInitialValue=ropod_kinmodel_param.C_SW(7)  SampleTime=Tsp  ShowErrorCodeOutput=on  ModelName=ROPOD_4Wheel_TdistZMPC_cntr  BlockId=ParamGet_ROPOD_4Wheel_TdistZMPC_cntr_2190
      settings: SourceProductName=Robotics System Toolbox  SourceProductBaseCode=RO
  Mux : Mux  Inputs=18
  Terminator{,1..17} (18 alike) : Terminator
  ropod_kin_param : Outport
  wires:
  Mux/1 -> ropod_kin_param/1
  Get Parameter/2 -> Terminator/1
  Get Parameter13/1 -> Mux/4
  Get Parameter15/2 -> Terminator15/1
  Get Parameter14/2 -> Terminator14/1
  Get Parameter16/1 -> Mux/7
  Get Parameter15/1 -> Mux/6
  Get Parameter11/1 -> Mux/2
  Get Parameter11/2 -> Terminator11/1
  Get Parameter16/2 -> Terminator16/1
  Get Parameter12/2 -> Terminator12/1
  Get Parameter12/1 -> Mux/3
  Get Parameter/1 -> Mux/1
  Get Parameter17/2 -> Terminator17/1
  Get Parameter13/2 -> Terminator13/1
  Get Parameter17/1 -> Mux/8
  Get Parameter14/1 -> Mux/5
  Get Parameter2/2 -> Terminator2/1
  Get Parameter2/1 -> Mux/10
  Get Parameter1/1 -> Mux/9
  Get Parameter1/2 -> Terminator1/1
  Get Parameter6/2 -> Terminator6/1
  Get Parameter6/1 -> Mux/14
  Get Parameter3/1 -> Mux/11
  Get Parameter5/2 -> Terminator5/1
  Get Parameter5/1 -> Mux/13
  Get Parameter4/1 -> Mux/12
  Get Parameter3/2 -> Terminator3/1
  Get Parameter4/2 -> Terminator4/1
  Get Parameter10/1 -> Mux/18
  Get Parameter10/2 -> Terminator10/1
  Get Parameter8/2 -> Terminator8/1
  Get Parameter7/2 -> Terminator7/1
  Get Parameter9/2 -> Terminator9/1
  Get Parameter7/1 -> Mux/15
  Get Parameter8/1 -> Mux/16
  Get Parameter9/1 -> Mux/17

== system ROPOD_4Wheel_TdistZMPC_cntr/ROS Smart wheels conf ==
  Bus Creator : BusCreator  Inputs=6
  Get Parameter : robotlib/Get Parameter  SourceLibraryInfo=This block requires Robotics System Toolbox  ParameterSource=Specify your own  ParameterName=/smart_wheels/enable  ParameterType=double  ParameterMaxArrayLength=16  ParameterInitialValue=sw_ini_enable  SampleTime=Tsp  ShowErrorCodeOutput=on  ModelName=ROPOD_4Wheel_TdistZMPC_cntr  BlockId=ParamGet_ROPOD_4Wheel_TdistZMPC_cntr_2213
      settings: SourceProductName=Robotics System Toolbox  SourceProductBaseCode=RO
  Get Parameter1 : robotlib/Get Parameter  SourceLibraryInfo=This block requires Robotics System Toolbox  ParameterSource=Specify your own  ParameterName=/smart_wheels/pivot_offs_sw1  ParameterType=double  ParameterMaxArrayLength=16  ParameterInitialValue=pivot_offs_sws(1)  SampleTime=Tsp  ShowErrorCodeOutput=on  ModelName=ROPOD_4Wheel_TdistZMPC_cntr  BlockId=ParamGet_ROPOD_4Wheel_TdistZMPC_cntr_2214
      settings: SourceProductName=Robotics System Toolbox  SourceProductBaseCode=RO
  Get Parameter2 : robotlib/Get Parameter  SourceLibraryInfo=This block requires Robotics System Toolbox  ParameterSource=Specify your own  ParameterName=/smart_wheels/max_current  ParameterType=double  ParameterMaxArrayLength=16  ParameterInitialValue=max_sw_current  SampleTime=Tsp  ShowErrorCodeOutput=on  ModelName=ROPOD_4Wheel_TdistZMPC_cntr  BlockId=ParamGet_ROPOD_4Wheel_TdistZMPC_cntr_2215
      settings: SourceProductName=Robotics System Toolbox  SourceProductBaseCode=RO
  Get Parameter3 : robotlib/Get Parameter  SourceLibraryInfo=This block requires Robotics System Toolbox  ParameterSource=Specify your own  ParameterName=/smart_wheels/pivot_offs_sw2  ParameterType=double  ParameterMaxArrayLength=16  ParameterInitialValue=pivot_offs_sws(2)  SampleTime=Tsp  ShowErrorCodeOutput=on  ModelName=ROPOD_4Wheel_TdistZMPC_cntr  BlockId=ParamGet_ROPOD_4Wheel_TdistZMPC_cntr_2216
      settings: SourceProductName=Robotics System Toolbox  SourceProductBaseCode=RO
  Get Parameter4 : robotlib/Get Parameter  SourceLibraryInfo=This block requires Robotics System Toolbox  ParameterSource=Specify your own  ParameterName=/smart_wheels/pivot_offs_sw3  ParameterType=double  ParameterMaxArrayLength=16  ParameterInitialValue=pivot_offs_sws(3)  SampleTime=Tsp  ShowErrorCodeOutput=on  ModelName=ROPOD_4Wheel_TdistZMPC_cntr  BlockId=ParamGet_ROPOD_4Wheel_TdistZMPC_cntr_2217
      settings: SourceProductName=Robotics System Toolbox  SourceProductBaseCode=RO
  Get Parameter5 : robotlib/Get Parameter  SourceLibraryInfo=This block requires Robotics System Toolbox  ParameterSource=Specify your own  ParameterName=/smart_wheels/pivot_offs_sw4  ParameterType=double  ParameterMaxArrayLength=16  ParameterInitialValue=pivot_offs_sws(4)  SampleTime=Tsp  ShowErrorCodeOutput=on  ModelName=ROPOD_4Wheel_TdistZMPC_cntr  BlockId=ParamGet_ROPOD_4Wheel_TdistZMPC_cntr_2218
      settings: SourceProductName=Robotics System Toolbox  SourceProductBaseCode=RO
  Terminator{,1..5} (6 alike) : Terminator
  sw_conf : Outport
  wires:
  Get Parameter/2 -> Terminator/1
  Get Parameter/1 -> Bus Creator/1  "enable"
  Bus Creator/1 -> sw_conf/1
  Get Parameter2/2 -> Terminator2/1
  Get Parameter2/1 -> Bus Creator/2  "max_current"
  Get Parameter1/1 -> Bus Creator/3  "pivot_offs_sw1"
  Get Parameter1/2 -> Terminator1/1
  Get Parameter3/2 -> Terminator3/1
  Get Parameter3/1 -> Bus Creator/4  "pivot_offs_sw2"
  Get Parameter4/2 -> Terminator4/1
  Get Parameter4/1 -> Bus Creator/5  "pivot_offs_sw3"
  Get Parameter5/2 -> Terminator5/1
  Get Parameter5/1 -> Bus Creator/6  "pivot_offs_sw4"

== system ROPOD_4Wheel_TdistZMPC_cntr/ROS base conf ==
  Bus Creator : BusCreator  Inputs=4
  Get Parameter : robotlib/Get Parameter  SourceLibraryInfo=This block requires Robotics System Toolbox  ParameterSource=Specify your own  ParameterName=/base_conf/max_acc_xy  ParameterType=double  ParameterMaxArrayLength=16  ParameterInitialValue=max_ropod_acc_xy  SampleTime=Tsp  ShowErrorCodeOutput=on  ModelName=ROPOD_4Wheel_TdistZMPC_cntr  BlockId=ParamGet_ROPOD_4Wheel_TdistZMPC_cntr_2237
      settings: SourceProductName=Robotics System Toolbox  SourceProductBaseCode=RO
  Get Parameter1 : robotlib/Get Parameter  SourceLibraryInfo=This block requires Robotics System Toolbox  ParameterSource=Specify your own  ParameterName=/base_conf/max_vel_xy  ParameterType=double  ParameterMaxArrayLength=16  ParameterInitialValue=max_ropod_vel_xy  SampleTime=Tsp  ShowErrorCodeOutput=on  ModelName=ROPOD_4Wheel_TdistZMPC_cntr  BlockId=ParamGet_ROPOD_4Wheel_TdistZMPC_cntr_2238
      settings: SourceProductName=Robotics System Toolbox  SourceProductBaseCode=RO
  Get Parameter2 : robotlib/Get Parameter  SourceLibraryInfo=This block requires Robotics System Toolbox  ParameterSource=Specify your own  ParameterName=/base_conf/max_acc_theta  ParameterType=double  ParameterMaxArrayLength=16  ParameterInitialValue=max_ropod_acc_theta  SampleTime=Tsp  ShowErrorCodeOutput=on  ModelName=ROPOD_4Wheel_TdistZMPC_cntr  BlockId=ParamGet_ROPOD_4Wheel_TdistZMPC_cntr_2239
      settings: SourceProductName=Robotics System Toolbox  SourceProductBaseCode=RO
  Get Parameter3 : robotlib/Get Parameter  SourceLibraryInfo=This block requires Robotics System Toolbox  ParameterSource=Specify your own  ParameterName=/base_conf/max_vel_theta  ParameterType=double  ParameterMaxArrayLength=16  ParameterInitialValue=max_ropod_vel_theta  SampleTime=Tsp  ShowErrorCodeOutput=on  ModelName=ROPOD_4Wheel_TdistZMPC_cntr  BlockId=ParamGet_ROPOD_4Wheel_TdistZMPC_cntr_2240
      settings: SourceProductName=Robotics System Toolbox  SourceProductBaseCode=RO
  Terminator{,1..3} (4 alike) : Terminator
  base_conf : Outport
  wires:
  Get Parameter/2 -> Terminator/1
  Get Parameter1/2 -> Terminator1/1
  Get Parameter/1 -> Bus Creator/2  "max_acc_xy"
  Get Parameter1/1 -> Bus Creator/1  "max_vel_xy"
  Bus Creator/1 -> base_conf/1
  Get Parameter2/2 -> Terminator2/1
  Get Parameter2/1 -> Bus Creator/4  "max_acc_theta"
  Get Parameter3/1 -> Bus Creator/3  "max_vel_theta"
  Get Parameter3/2 -> Terminator3/1

== system ROPOD_4Wheel_TdistZMPC_cntr/Subsystem ==
  state : Inport
  "[Fxp; Txp; Fyp Typ; Fxm; Txm; Fym; Tym] " : Inport  Port=2
  load_applied : Inport  Port=3
  Demux : Demux  Outputs=8
  Publish : robotlib/Publish  SourceLibraryInfo=This block requires Robotics System Toolbox  topicSource=Specify your own  topic=/ropod/wrench_left  messageType=geometry_msgs/WrenchStamped  messageQueueLength=1
      settings: SourceProductBaseCode=RO
  Publish1 : robotlib/Publish  SourceLibraryInfo=This block requires Robotics System Toolbox  topicSource=Specify your own  topic=/ropod/wrench_front  messageType=geometry_msgs/WrenchStamped  messageQueueLength=1
      settings: SourceProductBaseCode=RO
  Publish2 : robotlib/Publish  SourceLibraryInfo=This block requires Robotics System Toolbox  topicSource=Specify your own  topic=/ropod/wrench_back  messageType=geometry_msgs/WrenchStamped  messageQueueLength=1
      settings: SourceProductBaseCode=RO
  Publish3 : robotlib/Publish  SourceLibraryInfo=This block requires Robotics System Toolbox  topicSource=Specify your own  topic=/ropod/wrench_right  messageType=geometry_msgs/WrenchStamped  messageQueueLength=1
      settings: SourceProductBaseCode=RO
  Publish4 : robotlib/Publish  SourceLibraryInfo=This block requires Robotics System Toolbox  topicSource=Specify your own  topic=/ropod/LLCmode_Applied  messageType=std_msgs/UInt16  messageQueueLength=1
      settings: SourceProductBaseCode=RO
  Publish5 : robotlib/Publish  SourceLibraryInfo=This block requires Robotics System Toolbox  topicSource=Specify your own  topic=/ropod/load_attached_Applied  messageType=std_msgs/Bool  messageQueueLength=1
      settings: SourceProductBaseCode=RO
  Subsystem : Subsystem
  Subsystem1 : Subsystem
  Subsystem2 : Subsystem
  Subsystem3 : Subsystem
  Subsystem4 : Subsystem
  Subsystem5 : Subsystem
  wires:
  "[Fxp; Txp; Fyp Typ; Fxm; Txm; Fym; Tym] "/1 -> Demux/1
  Demux/1 -> Subsystem/1(In1)
  Demux/2 -> Subsystem/2(In2)
  Subsystem/1(Out1) -> Publish1/1
  Demux/3 -> Subsystem1/1(In1)
  Demux/4 -> Subsystem1/2(In2)
  Demux/5 -> Subsystem2/1(In1)
  Demux/6 -> Subsystem2/2(In2)
  Demux/7 -> Subsystem3/1(In1)
  Demux/8 -> Subsystem3/2(In2)
  Subsystem1/1(Out1) -> Publish/1
  Subsystem2/1(Out1) -> Publish2/1
  Subsystem3/1(Out1) -> Publish3/1
  state/1 -> Subsystem4/1(In1)
  Subsystem4/1(Out1) -> Publish4/1
  load_applied/1 -> Subsystem5/1(In1)
  Subsystem5/1(Out1) -> Publish5/1

== system ROPOD_4Wheel_TdistZMPC_cntr/Non-ROS Ropod Controller/Odometry and Measurement model 4SW ==
  note: This output is only useful when using ros
      | This data is fed to /odom/pose
  note: This part is in global coordinates
  note: This part is in local coordinates
  param_in : Inport
  dvarphi : Inport  Port=2
  delta : Inport  Port=3
  Discrete-Time Integrator : DiscreteIntegrator  InitialConditionSetting=State (most efficient)  SampleTime=Ts  ICPrevOutput=DiscIntNeverNeededParam  ICPrevScaledInput=DiscIntNeverNeededParam
  Jqwl_matrix : MATLAB Function  TreatAsAtomicUnit=on
  Product3 : Product  Multiplication=Matrix(*)
  Selector3 : Selector  InputPortWidth=3  IndexOptions=Index vector (dialog)  Indices=3  OutputSizes=1
  Signal Specification : SignalSpecification  Dimensions=[3 1]
  pos_rot_matrix : MATLAB Function  TreatAsAtomicUnit=on
  odom_robot_pose : Outport
  odom_robot_twist : Outport  Port=2
  wires:
  Product3/1 -> Signal Specification/1
  param_in/1 -> Jqwl_matrix/1(ropod_kinmodel_param_vec)
  delta/1 -> Jqwl_matrix/2(delta)
  Jqwl_matrix/1(Jqwl) -> Product3/1
  dvarphi/1 -> Product3/2
  Signal Specification/1 -> pos_rot_matrix/1(dqr_loc), odom_robot_twist/1
  Selector3/1 -> pos_rot_matrix/2(theta_odom)
  pos_rot_matrix/1(dqr_glb) -> Discrete-Time Integrator/1
  Discrete-Time Integrator/1 -> odom_robot_pose/1, Selector3/1

== system ROPOD_4Wheel_TdistZMPC_cntr/Non-ROS Ropod Controller/ROPOD 4SW TORQUE_MODE ==
  sw_conf : Inport
  intialization : Inport  Port=2
  varphi_tau_setp : Inport  Port=3
  Bus Creator : BusCreator  Inputs=4
  Display1 : Display
  ECAT_Interface : SOEM_EtherCAT_Lib/ECAT_Interface  Priority=0  IFINTERFACE=eth0  TS=Ts
      settings: SourceProductName=SOEM_EtherCAT_Lib
  Gain1 : Gain  OutDataTypeStr=double
  Initialization switch : Subsystem
  ROPOD_4Wheel_sens : Subsystem
  ROPOD_4Wheel_torque_cmd : Subsystem
  Smart_Wheel_1 : Subsystem
  Smart_Wheel_2 : Subsystem
  Smart_Wheel_3 : Subsystem
  Smart_Wheel_4 : Subsystem
  Subsystem : Subsystem
  empywheel : Subsystem  Commented=on
  dvarphi : Outport
  delta : Outport  Port=2
  ddelta : Outport  Port=3
  SW_sens : Outport  Port=4
  wires:
  ROPOD_4Wheel_sens/2(delta) -> delta/1
  ROPOD_4Wheel_sens/1(dvarphi) -> dvarphi/1
  ECAT_Interface/1 -> Gain1/1
  Gain1/1 -> Display1/1
  ROPOD_4Wheel_sens/3(ddelta) -> ddelta/1
  ROPOD_4Wheel_torque_cmd/4(SW4_cmd) -> Smart_Wheel_4/1(SW4_cmd)
  ROPOD_4Wheel_torque_cmd/1(SW1_cmd) -> Smart_Wheel_1/1(SW1_cmd)
  ROPOD_4Wheel_torque_cmd/3(SW3_cmd) -> Smart_Wheel_3/1(SW3_cmd)
  sw_conf/1 -> ROPOD_4Wheel_torque_cmd/1(sw_conf), ROPOD_4Wheel_sens/2(sw_conf)
  ROPOD_4Wheel_torque_cmd/2(SW2_cmd) -> Smart_Wheel_2/1(SW2_cmd)
  Smart_Wheel_1/1(SW1_sens) -> Bus Creator/1, ROPOD_4Wheel_sens/3(SW1_sens)  "SW1_sens"
  Smart_Wheel_4/1(SW4_sens) -> ROPOD_4Wheel_sens/6(SW4_sens), Bus Creator/4  "SW4_sens"
  Smart_Wheel_2/1(SW2_sens) -> ROPOD_4Wheel_sens/4(SW2_sens), Bus Creator/2  "SW2_sens"
  Smart_Wheel_3/1(SW3_sens) -> ROPOD_4Wheel_sens/5(SW3_sens), Bus Creator/3  "SW3_sens"
  Bus Creator/1 -> SW_sens/1
  Initialization switch/1(cntr_mode) -> ROPOD_4Wheel_torque_cmd/2(cntr_mode)
  Initialization switch/2(wheel_setp) -> ROPOD_4Wheel_torque_cmd/3(wheel_setp)
  Subsystem/1(varphi_curr_setp) -> Initialization switch/2(In2)
  varphi_tau_setp/1 -> Subsystem/1(varphi_tau_setp)
  intialization/1 -> ROPOD_4Wheel_sens/1(disable), Initialization switch/1(vel_mode_enable)

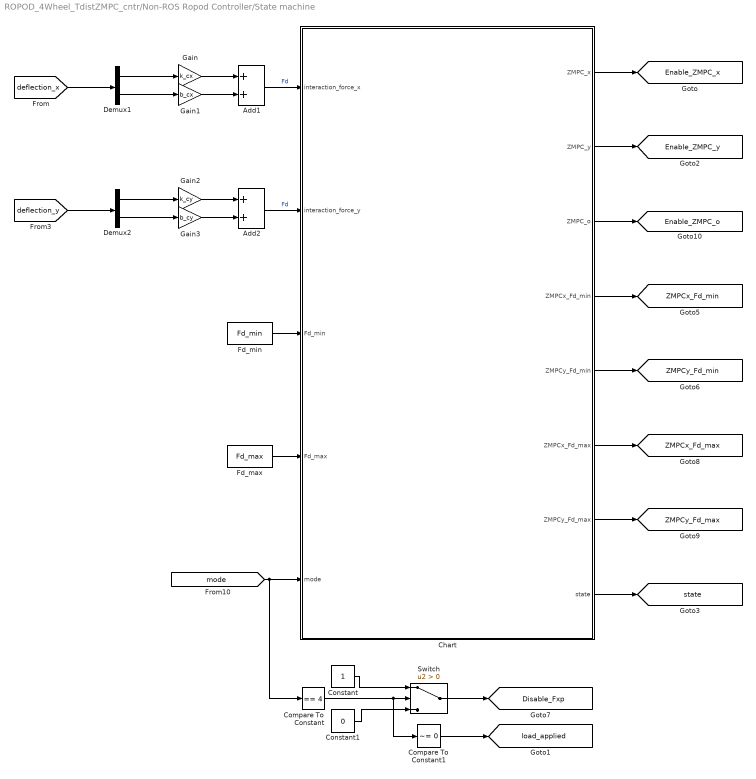
== system ROPOD_4Wheel_TdistZMPC_cntr/Non-ROS Ropod Controller/State machine ==
  Add1 : Sum
  Add2 : Sum
  Chart : Stateflow chart  TreatAsAtomicUnit=on
  Compare To Constant : simulink/Logic and Bit Operations/Compare To Constant  relop===  const=4  OutDataTypeStr=boolean
  Compare To Constant1 : simulink/Logic and Bit Operations/Compare To Constant  relop=~=  const=0  OutDataTypeStr=boolean
  Constant : Constant
  Constant1 : Constant  Value=0
  Demux1 : Demux  Outputs=2
  Demux2 : Demux  Outputs=2
  Fd_max : Constant  Value=Fd_max
  Fd_min : Constant  Value=Fd_min
  Gain : Gain  Gain=k_cx
  Gain1 : Gain  Gain=b_cx
  Gain2 : Gain  Gain=k_cy
  Gain3 : Gain  Gain=b_cy
  Switch : Switch  Criteria=u2 > Threshold
  tag scope: Disable_Fxp=global, Enable_ZMPC_o=global, Enable_ZMPC_x=global, Enable_ZMPC_y=global, ZMPCx_Fd_max=global, ZMPCx_Fd_min=global, ZMPCy_Fd_max=global, ZMPCy_Fd_min=global, load_applied=global, state=global
  wires:
  Chart/2(ZMPC_y) -> [Enable_ZMPC_y]
  Demux1/1 -> Gain/1
  [deflection_y] -> Demux2/1
  Gain/1 -> Add1/1
  Add1/1 -> Chart/1(interaction_force_x)  "Fd"
  Add2/1 -> Chart/2(interaction_force_y)  "Fd"
  Fd_min/1 -> Chart/3(Fd_min)
  Demux2/1 -> Gain2/1
  [deflection_x] -> Demux1/1
  Gain3/1 -> Add2/2
  Demux2/2 -> Gain3/1
  Chart/1(ZMPC_x) -> [Enable_ZMPC_x]
  Gain1/1 -> Add1/2
  Demux1/2 -> Gain1/1
  Gain2/1 -> Add2/1
  [mode] -> Compare To Constant/1, Chart/5(mode)
  Chart/4(ZMPCx_Fd_min) -> [ZMPCx_Fd_min]
  Chart/5(ZMPCy_Fd_min) -> [ZMPCy_Fd_min]
  Fd_max/1 -> Chart/4(Fd_max)
  Chart/7(ZMPCy_Fd_max) -> [ZMPCy_Fd_max]
  Chart/6(ZMPCx_Fd_max) -> [ZMPCx_Fd_max]
  Chart/3(ZMPC_o) -> [Enable_ZMPC_o]
  Chart/8(state) -> [state]
  Compare To Constant/1 -> Compare To Constant1/1, Switch/2
  Constant1/1 -> Switch/3
  Constant/1 -> Switch/1
  Switch/1 -> [Disable_Fxp]
  Compare To Constant1/1 -> [load_applied]

== system ROPOD_4Wheel_TdistZMPC_cntr/Non-ROS Ropod Controller/State machine1 ==
  Add1 : Sum
  Add2 : Sum
  Chart : Stateflow chart  TreatAsAtomicUnit=on
  Compare To Constant : simulink/Logic and Bit Operations/Compare To Constant  relop===  const=4  OutDataTypeStr=boolean
  Constant : Constant
  Constant1 : Constant  Value=0
  Demux1 : Demux  Outputs=2
  Demux2 : Demux  Outputs=2
  Fd_max : Constant  Value=Fd_max
  Fd_min : Constant  Value=Fd_min
  Gain : Gain  Gain=k_cx
  Gain1 : Gain  Gain=b_cx
  Gain2 : Gain  Gain=k_cy
  Gain3 : Gain  Gain=b_cy
  Switch : Switch  Criteria=u2 > Threshold
  tag scope: Disable_Fxp=global, Enable_ZMPC_o=global, Enable_ZMPC_x=global, Enable_ZMPC_y=global, ZMPCx_Fd_max=global, ZMPCx_Fd_min=global, ZMPCy_Fd_max=global, ZMPCy_Fd_min=global, state=global
  wires:
  Chart/2(ZMPC_y) -> [Enable_ZMPC_y]
  Demux1/1 -> Gain/1
  [deflection_y] -> Demux2/1
  Gain/1 -> Add1/1
  Add1/1 -> Chart/1(interaction_force_x)  "Fd"
  Add2/1 -> Chart/2(interaction_force_y)  "Fd"
  Fd_min/1 -> Chart/3(Fd_min)
  Demux2/1 -> Gain2/1
  [deflection_x] -> Demux1/1
  Gain3/1 -> Add2/2
  Demux2/2 -> Gain3/1
  Chart/1(ZMPC_x) -> [Enable_ZMPC_x]
  Gain1/1 -> Add1/2
  Demux1/2 -> Gain1/1
  Gain2/1 -> Add2/1
  [mode] -> Compare To Constant/1, Chart/5(mode)
  Chart/4(ZMPCx_Fd_min) -> [ZMPCx_Fd_min]
  Chart/5(ZMPCy_Fd_min) -> [ZMPCy_Fd_min]
  Fd_max/1 -> Chart/4(Fd_max)
  Chart/7(ZMPCy_Fd_max) -> [ZMPCy_Fd_max]
  Chart/6(ZMPCx_Fd_max) -> [ZMPCx_Fd_max]
  Chart/3(ZMPC_o) -> [Enable_ZMPC_o]
  Chart/8(state) -> [state]
  Switch/1 -> [Disable_Fxp]
  Compare To Constant/1 -> Switch/2
  Constant1/1 -> Switch/3
  Constant/1 -> Switch/1

== system ROPOD_4Wheel_TdistZMPC_cntr/Non-ROS Ropod Controller/Subsystem ==
  In2 : Inport
  Constant1 : Constant  Value=0
  Logical Operator : Logic  Operator=OR  Inputs=3  AllPortsSameDT=off  OutDataTypeStr=boolean
  Switch1 : Switch  Criteria=u2 > Threshold
  Out2 : Outport
  wires:
  [Enable_ZMPC_o] -> Logical Operator/3
  Constant1/1 -> Switch1/1
  Logical Operator/1 -> Switch1/2
  [Enable_ZMPC_x] -> Logical Operator/1
  Switch1/1 -> Out2/1
  In2/1 -> Switch1/3
  [Enable_ZMPC_y] -> Logical Operator/2
